simulink model "MotoTron_validation_IO_model_integration"  (R2018a)
settings: Solver=FixedStepDiscrete  StartTime=0.0  StopTime=10.0  RelTol=1e-3  EnableMultiTasking=on
undefined symbols (not defined in the file or in its folder): ECU565, motohawk_build_version, motohawk_trunc_name, motohawk_vardec_path
libraries: MotoHawk_lib x73, simulink x16, motohawk_examples_lib x1
(part 2 of 2)

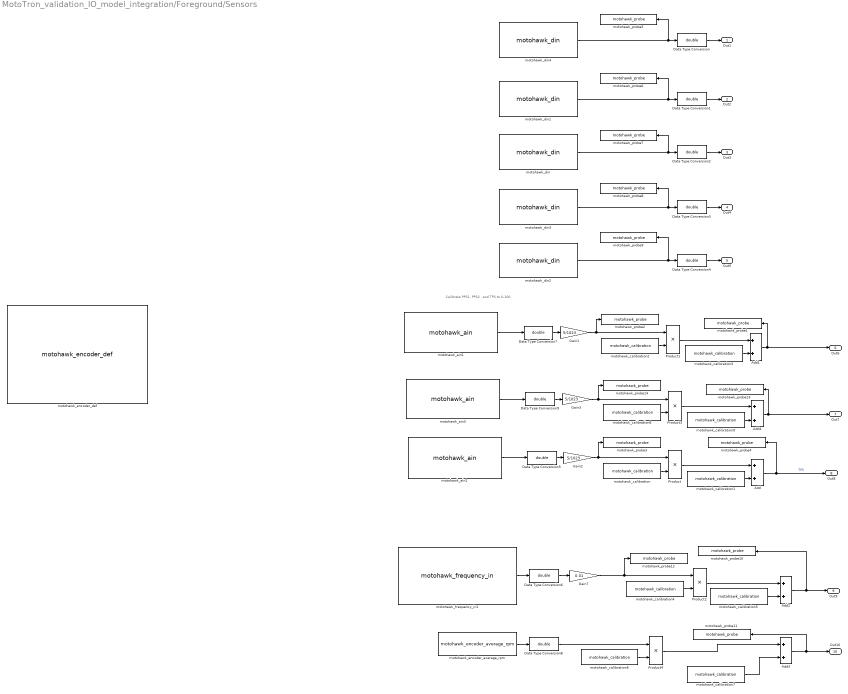
== system MotoTron_validation_IO_model_integration/Foreground/Sensors ==
  note: Calibrate PPS1, PPS2 , and TPS to 0-100
  Add{,1..4} (5 alike) : Sum
  Data Type Conversion{,1..9} (10 alike) : DataTypeConversion  OutDataTypeStr=double
  Gain1 : Gain  Gain=5/1023
  Gain2 : Gain  Gain=5/1023
  Gain3 : Gain  Gain=5/1023
  Gain7 : Gain  Gain=0.01
  Product{,1..4} (5 alike) : Product  RndMeth=Zero
  motohawk_ain1 : MotoHawk_lib/Analog I//O Blocks/motohawk_ain  res_name='PPS1'  text_resource=AN2M  code_resource=NONE  val_resource=-1  target=ECU565-128  resource_enum_str=(None)=-1,ECUP=53,DRVP=54,XDRP=55,AN1M=56,AN2M=57,AN3M=58,AN4M=59,AN5M=60,AN6M=61,AN7M=62,AN8M=63,AN9M=64,AN10M=65,AN11M=66,AN12M=67,AN13M=68,AN14M=69,AN15M=70,AN16M=71,AN17M=72,AN18M=73,AN19M=74,AN20M=75,AN21M=76,AN22M=77,AN23M=78,AN24M=79,AN25M=80,AN26M=81,AN27M=82,AN28M=83,AN29M=84,AN30M=85,AN31M=86,AN32M=87,AN33M=88,AN34M=89,O2A=90,O2B=91,XDRP_B=92,REF_14V=143  altref=5V Reference  typ=uint16  num_adc_bits=10  use_stat=off  use_vardec=off  nam='RTD1_MW'  read_level=1  write_level=1  group='System | I/O Pins | Inputs Config'
      settings: SourceProductName=MotoHawk
  motohawk_ain2 : MotoHawk_lib/Analog I//O Blocks/motohawk_ain  res_name='TPS'  text_resource=AN4M  code_resource=NONE  val_resource=-1  target=ECU565-128  resource_enum_str=(None)=-1,ECUP=53,DRVP=54,XDRP=55,AN1M=56,AN2M=57,AN3M=58,AN4M=59,AN5M=60,AN6M=61,AN7M=62,AN8M=63,AN9M=64,AN10M=65,AN11M=66,AN12M=67,AN13M=68,AN14M=69,AN15M=70,AN16M=71,AN17M=72,AN18M=73,AN19M=74,AN20M=75,AN21M=76,AN22M=77,AN23M=78,AN24M=79,AN25M=80,AN26M=81,AN27M=82,AN28M=83,AN29M=84,AN30M=85,AN31M=86,AN32M=87,AN33M=88,AN34M=89,O2A=90,O2B=91,XDRP_B=92,REF_14V=143  altref=5V Reference  typ=uint16  num_adc_bits=10  use_stat=off  use_vardec=off  nam='RTD1_MW'  read_level=1  write_level=1  group='System | I/O Pins | Inputs Config'
      settings: SourceProductName=MotoHawk
  motohawk_ain3 : MotoHawk_lib/Analog I//O Blocks/motohawk_ain  res_name='PPS2'  text_resource=AN3M  code_resource=NONE  val_resource=-1  target=ECU565-128  resource_enum_str=(None)=-1,ECUP=53,DRVP=54,XDRP=55,AN1M=56,AN2M=57,AN3M=58,AN4M=59,AN5M=60,AN6M=61,AN7M=62,AN8M=63,AN9M=64,AN10M=65,AN11M=66,AN12M=67,AN13M=68,AN14M=69,AN15M=70,AN16M=71,AN17M=72,AN18M=73,AN19M=74,AN20M=75,AN21M=76,AN22M=77,AN23M=78,AN24M=79,AN25M=80,AN26M=81,AN27M=82,AN28M=83,AN29M=84,AN30M=85,AN31M=86,AN32M=87,AN33M=88,AN34M=89,O2A=90,O2B=91,XDRP_B=92,REF_14V=143  altref=5V Reference  typ=uint16  num_adc_bits=10  use_stat=off  use_vardec=off  nam='RTD1_MW'  read_level=1  write_level=1  group='System | I/O Pins | Inputs Config'
      settings: SourceProductName=MotoHawk
  motohawk_calibration : MotoHawk_lib/Calibration & Probing Blocks/motohawk_calibration  nam='TPS_Gain'  val=1  storage=Calibration  show_more=on  name_source=Use Parameter  data_type=Inherit from 'Default Value'  read_level=1  write_level=1  ovr_cals=off  view_as=Number  enum_struct={'Disabled', 'Enabled'}  vector_style=Wide Row  use_help_units=off  help=''  units=''  use_header_enum=off  row_header_enum={}  col_header_enum={}  use_min_max=off  min_val=-inf  max_val=inf  use_precision=off  precision=''  gain=1  offset=0  exp=1  use_mototune_group=off  mototune_group=motohawk_vardec_path(gcb)  data_stores=motohawk_sfun_calibration_data_stores
      settings: SourceProductName=MotoHawk
  motohawk_calibration1 : MotoHawk_lib/Calibration & Probing Blocks/motohawk_calibration  nam='TPS_Offset'  val=0  storage=Calibration  show_more=on  name_source=Use Parameter  data_type=Inherit from 'Default Value'  read_level=1  write_level=1  ovr_cals=off  view_as=Number  enum_struct={'Disabled', 'Enabled'}  vector_style=Wide Row  use_help_units=off  help=''  units=''  use_header_enum=off  row_header_enum={}  col_header_enum={}  use_min_max=off  min_val=-inf  max_val=inf  use_precision=off  precision=''  gain=1  offset=0  exp=1  use_mototune_group=off  mototune_group=motohawk_vardec_path(gcb)  data_stores=motohawk_sfun_calibration_data_stores
      settings: SourceProductName=MotoHawk
  motohawk_calibration2 : MotoHawk_lib/Calibration & Probing Blocks/motohawk_calibration  nam='PPS1_Gain'  val=1  storage=Calibration  show_more=on  name_source=Use Parameter  data_type=Inherit from 'Default Value'  read_level=1  write_level=1  ovr_cals=off  view_as=Number  enum_struct={'Disabled', 'Enabled'}  vector_style=Wide Row  use_help_units=off  help=''  units=''  use_header_enum=off  row_header_enum={}  col_header_enum={}  use_min_max=off  min_val=-inf  max_val=inf  use_precision=off  precision=''  gain=1  offset=0  exp=1  use_mototune_group=off  mototune_group=motohawk_vardec_path(gcb)  data_stores=motohawk_sfun_calibration_data_stores
      settings: SourceProductName=MotoHawk
  motohawk_calibration3 : MotoHawk_lib/Calibration & Probing Blocks/motohawk_calibration  nam='PPS1_Offset'  val=0  storage=Calibration  show_more=on  name_source=Use Parameter  data_type=Inherit from 'Default Value'  read_level=1  write_level=1  ovr_cals=off  view_as=Number  enum_struct={'Disabled', 'Enabled'}  vector_style=Wide Row  use_help_units=off  help=''  units=''  use_header_enum=off  row_header_enum={}  col_header_enum={}  use_min_max=off  min_val=-inf  max_val=inf  use_precision=off  precision=''  gain=1  offset=0  exp=1  use_mototune_group=off  mototune_group=motohawk_vardec_path(gcb)  data_stores=motohawk_sfun_calibration_data_stores
      settings: SourceProductName=MotoHawk
  motohawk_calibration4 : MotoHawk_lib/Calibration & Probing Blocks/motohawk_calibration  nam='Vehicle_Speed_Gain'  val=1  storage=Calibration  show_more=on  name_source=Use Parameter  data_type=Inherit from 'Default Value'  read_level=1  write_level=1  ovr_cals=off  view_as=Number  enum_struct={'Disabled', 'Enabled'}  vector_style=Wide Row  use_help_units=off  help=''  units=''  use_header_enum=off  row_header_enum={}  col_header_enum={}  use_min_max=off  min_val=-inf  max_val=inf  use_precision=off  precision=''  gain=1  offset=0  exp=1  use_mototune_group=off  mototune_group=motohawk_vardec_path(gcb)  data_stores=motohawk_sfun_calibration_data_stores
      settings: SourceProductName=MotoHawk
  motohawk_calibration5 : MotoHawk_lib/Calibration & Probing Blocks/motohawk_calibration  nam='Vehicle_Speed_Offset'  val=0  storage=Calibration  show_more=on  name_source=Use Parameter  data_type=Inherit from 'Default Value'  read_level=1  write_level=1  ovr_cals=off  view_as=Number  enum_struct={'Disabled', 'Enabled'}  vector_style=Wide Row  use_help_units=off  help=''  units=''  use_header_enum=off  row_header_enum={}  col_header_enum={}  use_min_max=off  min_val=-inf  max_val=inf  use_precision=off  precision=''  gain=1  offset=0  exp=1  use_mototune_group=off  mototune_group=motohawk_vardec_path(gcb)  data_stores=motohawk_sfun_calibration_data_stores
      settings: SourceProductName=MotoHawk
  motohawk_calibration6 : MotoHawk_lib/Calibration & Probing Blocks/motohawk_calibration  nam='Engine_RPM_Gain'  val=1  storage=Calibration  show_more=on  name_source=Use Parameter  data_type=Inherit from 'Default Value'  read_level=1  write_level=1  ovr_cals=off  view_as=Number  enum_struct={'Disabled', 'Enabled'}  vector_style=Wide Row  use_help_units=off  help=''  units=''  use_header_enum=off  row_header_enum={}  col_header_enum={}  use_min_max=off  min_val=-inf  max_val=inf  use_precision=off  precision=''  gain=1  offset=0  exp=1  use_mototune_group=off  mototune_group=motohawk_vardec_path(gcb)  data_stores=motohawk_sfun_calibration_data_stores
      settings: SourceProductName=MotoHawk
  motohawk_calibration7 : MotoHawk_lib/Calibration & Probing Blocks/motohawk_calibration  nam='Engine_RPM_Offset'  val=0  storage=Calibration  show_more=on  name_source=Use Parameter  data_type=Inherit from 'Default Value'  read_level=1  write_level=1  ovr_cals=off  view_as=Number  enum_struct={'Disabled', 'Enabled'}  vector_style=Wide Row  use_help_units=off  help=''  units=''  use_header_enum=off  row_header_enum={}  col_header_enum={}  use_min_max=off  min_val=-inf  max_val=inf  use_precision=off  precision=''  gain=1  offset=0  exp=1  use_mototune_group=off  mototune_group=motohawk_vardec_path(gcb)  data_stores=motohawk_sfun_calibration_data_stores
      settings: SourceProductName=MotoHawk
  motohawk_calibration8 : MotoHawk_lib/Calibration & Probing Blocks/motohawk_calibration  nam='PPS2_Gain'  val=1  storage=Calibration  show_more=on  name_source=Use Parameter  data_type=Inherit from 'Default Value'  read_level=1  write_level=1  ovr_cals=off  view_as=Number  enum_struct={'Disabled', 'Enabled'}  vector_style=Wide Row  use_help_units=off  help=''  units=''  use_header_enum=off  row_header_enum={}  col_header_enum={}  use_min_max=off  min_val=-inf  max_val=inf  use_precision=off  precision=''  gain=1  offset=0  exp=1  use_mototune_group=off  mototune_group=motohawk_vardec_path(gcb)  data_stores=motohawk_sfun_calibration_data_stores
      settings: SourceProductName=MotoHawk
  motohawk_calibration9 : MotoHawk_lib/Calibration & Probing Blocks/motohawk_calibration  nam='PPS2_Offset'  val=0  storage=Calibration  show_more=on  name_source=Use Parameter  data_type=Inherit from 'Default Value'  read_level=1  write_level=1  ovr_cals=off  view_as=Number  enum_struct={'Disabled', 'Enabled'}  vector_style=Wide Row  use_help_units=off  help=''  units=''  use_header_enum=off  row_header_enum={}  col_header_enum={}  use_min_max=off  min_val=-inf  max_val=inf  use_precision=off  precision=''  gain=1  offset=0  exp=1  use_mototune_group=off  mototune_group=motohawk_vardec_path(gcb)  data_stores=motohawk_sfun_calibration_data_stores
      settings: SourceProductName=MotoHawk
  motohawk_din : MotoHawk_lib/Digital I//O Blocks/motohawk_din  resource_name='Motor_On_Switch'  text_resource=AN6M  code_resource=NONE  val_resource=-1  target=ECU565-128  resource_enum_str=(None)=-1,AN1M=56,AN2M=57,AN3M=58,AN4M=59,AN5M=60,AN6M=61,AN7M=62,AN8M=63,AN9M=64,AN10M=65,AN11M=66,AN12M=67,AN13M=68,AN14M=69,AN15M=70,AN16M=71,AN17M=72,AN18M=73,AN19M=74,AN20M=75,AN21M=76,AN22M=77,AN23M=78,AN24M=79,AN25M=80,AN26M=81,AN27M=82,AN28M=83,AN29M=84,AN30M=85,AN31M=86,AN32M=87,AN33M=88,AN34M=89,O2A=90,O2B=91,DG1M=93,DG2M=94,DG3M=95,DG4M=96,DG5M=102,DG6M=103,DG7M=104,SPD1=105,SPD2=106,DG8M=111  pullup=Strong  use_stat=off  use_vardec=off  nam='DIN'  read_level=1  write_level=1  group='System | I/O Pins | Inputs Config'
      settings: SourceProductName=MotoHawk
  motohawk_din1 : MotoHawk_lib/Digital I//O Blocks/motohawk_din  resource_name='Engine_On_Switch'  text_resource=AN5M  code_resource=NONE  val_resource=-1  target=ECU565-128  resource_enum_str=(None)=-1,AN1M=56,AN2M=57,AN3M=58,AN4M=59,AN5M=60,AN6M=61,AN7M=62,AN8M=63,AN9M=64,AN10M=65,AN11M=66,AN12M=67,AN13M=68,AN14M=69,AN15M=70,AN16M=71,AN17M=72,AN18M=73,AN19M=74,AN20M=75,AN21M=76,AN22M=77,AN23M=78,AN24M=79,AN25M=80,AN26M=81,AN27M=82,AN28M=83,AN29M=84,AN30M=85,AN31M=86,AN32M=87,AN33M=88,AN34M=89,O2A=90,O2B=91,DG1M=93,DG2M=94,DG3M=95,DG4M=96,DG5M=102,DG6M=103,DG7M=104,SPD1=105,SPD2=106,DG8M=111  pullup=Strong  use_stat=off  use_vardec=off  nam='DIN'  read_level=1  write_level=1  group='System | I/O Pins | Inputs Config'
      settings: SourceProductName=MotoHawk
  motohawk_din2 : MotoHawk_lib/Digital I//O Blocks/motohawk_din  resource_name='Reverse_Switch'  text_resource=AN8M  code_resource=NONE  val_resource=-1  target=ECU565-128  resource_enum_str=(None)=-1,AN1M=56,AN2M=57,AN3M=58,AN4M=59,AN5M=60,AN6M=61,AN7M=62,AN8M=63,AN9M=64,AN10M=65,AN11M=66,AN12M=67,AN13M=68,AN14M=69,AN15M=70,AN16M=71,AN17M=72,AN18M=73,AN19M=74,AN20M=75,AN21M=76,AN22M=77,AN23M=78,AN24M=79,AN25M=80,AN26M=81,AN27M=82,AN28M=83,AN29M=84,AN30M=85,AN31M=86,AN32M=87,AN33M=88,AN34M=89,O2A=90,O2B=91,DG1M=93,DG2M=94,DG3M=95,DG4M=96,DG5M=102,DG6M=103,DG7M=104,SPD1=105,SPD2=106,DG8M=111  pullup=Strong  use_stat=off  use_vardec=off  nam='DIN'  read_level=1  write_level=1  group='System | I/O Pins | Inputs Config'
      settings: SourceProductName=MotoHawk
  motohawk_din3 : MotoHawk_lib/Digital I//O Blocks/motohawk_din  resource_name='Forward_Switch'  text_resource=AN7M  code_resource=NONE  val_resource=-1  target=ECU565-128  resource_enum_str=(None)=-1,AN1M=56,AN2M=57,AN3M=58,AN4M=59,AN5M=60,AN6M=61,AN7M=62,AN8M=63,AN9M=64,AN10M=65,AN11M=66,AN12M=67,AN13M=68,AN14M=69,AN15M=70,AN16M=71,AN17M=72,AN18M=73,AN19M=74,AN20M=75,AN21M=76,AN22M=77,AN23M=78,AN24M=79,AN25M=80,AN26M=81,AN27M=82,AN28M=83,AN29M=84,AN30M=85,AN31M=86,AN32M=87,AN33M=88,AN34M=89,O2A=90,O2B=91,DG1M=93,DG2M=94,DG3M=95,DG4M=96,DG5M=102,DG6M=103,DG7M=104,SPD1=105,SPD2=106,DG8M=111  pullup=Strong  use_stat=off  use_vardec=off  nam='DIN'  read_level=1  write_level=1  group='System | I/O Pins | Inputs Config'
      settings: SourceProductName=MotoHawk
  motohawk_din4 : MotoHawk_lib/Digital I//O Blocks/motohawk_din  resource_name='Crank_Switch'  text_resource=AN9M  code_resource=NONE  val_resource=-1  target=ECU565-128  resource_enum_str=(None)=-1,AN1M=56,AN2M=57,AN3M=58,AN4M=59,AN5M=60,AN6M=61,AN7M=62,AN8M=63,AN9M=64,AN10M=65,AN11M=66,AN12M=67,AN13M=68,AN14M=69,AN15M=70,AN16M=71,AN17M=72,AN18M=73,AN19M=74,AN20M=75,AN21M=76,AN22M=77,AN23M=78,AN24M=79,AN25M=80,AN26M=81,AN27M=82,AN28M=83,AN29M=84,AN30M=85,AN31M=86,AN32M=87,AN33M=88,AN34M=89,O2A=90,O2B=91,DG1M=93,DG2M=94,DG3M=95,DG4M=96,DG5M=102,DG6M=103,DG7M=104,SPD1=105,SPD2=106,DG8M=111  pullup=Strong  use_stat=off  use_vardec=off  nam='DIN'  read_level=1  write_level=1  group='System | I/O Pins | Inputs Config'
      settings: SourceProductName=MotoHawk
  motohawk_encoder_average_rpm : MotoHawk_lib/Encoder Blocks/motohawk_encoder_average_rpm  resolution=1
      settings: SourceProductName=MotoHawk
  motohawk_encoder_def : MotoHawk_lib/Encoder Blocks/motohawk_encoder_def  encoder_type=36 Minus 1 - 4-Stroke - No CAM  interface=Digital Crank  sync=Falling Edge  crnkpullup=Weak Pullup  camsync=Rising Edge  campullup=Weak Pullup  angle_offset=0  sec_tdcoffset=0  cam_delay=0  teeth_after_cam=-1  ignore_teeth=0  ignore_delay=0  angles=[0 360 180 540]  cnk_align_with_cam=off  adaptive_vr_cnk=off  adaptive_vr_cam=on  cal_cylinders=on  max_cylinders=8  num_cylinders=1  read_level=1  write_level=1  ovr_cals=on  group='System | Encoder'
      settings: SourceProductName=MotoHawk
  motohawk_frequency_in1 : MotoHawk_lib/Advanced Digital I//O/motohawk_frequency_in  res_name='Vehicle_Speed'  text_resource=SPD1  code_resource=NONE  val_resource=-1  target=ECU565-128  resource_enum_str=(None)=-1,DG1M=93,DG2M=94,DG3M=95,DG4M=96,DG5M=102,DG6M=103,DG7M=104,SPD1=105,SPD2=106,DG8M=111  edge=Rising Edge  alias=Enabled  min_freq=0  sig=Digital Input  ipwm=No Duty Cycle Measurement  show_newness_status=off  itrig=off  Nmax=10  use_avg=off  avg_mode=Fixed Interval  fixed_avg_pulses=2  use_vardec=off  use_cal=off  nam='FreqInPin'  read_level=1  write_level=1  group='System | I/O Pins | Inputs Config'  cal_group='System | I/O Pins | Frequency In Config'
      settings: SourceProductName=MotoHawk
  motohawk_probe1 : MotoHawk_lib/Calibration & Probing Blocks/motohawk_probe  nam='PPS1'  show_more=off  name_source=Use Parameter  read_level=1  view_as=Number  enum_struct={'Disabled', 'Enabled'}  vector_style=Wide Row  use_help_units=off  help=''  units=''  use_header_enum=off  row_header_enum={}  col_header_enum={}  use_min_max=off  min_val=-inf  max_val=inf  use_precision=off  precision=''  gain=1  offset=0  exp=1  use_mototune_group=off  mototune_group=motohawk_vardec_path(gcb)
      settings: SourceProductName=MotoHawk
  motohawk_probe10 : MotoHawk_lib/Calibration & Probing Blocks/motohawk_probe  nam='Vehicle_Speed'  show_more=off  name_source=Use Parameter  read_level=1  view_as=Number  enum_struct={'Disabled', 'Enabled'}  vector_style=Wide Row  use_help_units=off  help=''  units=''  use_header_enum=off  row_header_enum={}  col_header_enum={}  use_min_max=off  min_val=-inf  max_val=inf  use_precision=off  precision=''  gain=1  offset=0  exp=1  use_mototune_group=off  mototune_group=motohawk_vardec_path(gcb)
      settings: SourceProductName=MotoHawk
  motohawk_probe11 : MotoHawk_lib/Calibration & Probing Blocks/motohawk_probe  nam='Engine_RPM'  show_more=off  name_source=Use Parameter  read_level=1  view_as=Number  enum_struct={'Disabled', 'Enabled'}  vector_style=Wide Row  use_help_units=off  help=''  units=''  use_header_enum=off  row_header_enum={}  col_header_enum={}  use_min_max=off  min_val=-inf  max_val=inf  use_precision=off  precision=''  gain=1  offset=0  exp=1  use_mototune_group=off  mototune_group=motohawk_vardec_path(gcb)
      settings: SourceProductName=MotoHawk
  motohawk_probe12 : MotoHawk_lib/Calibration & Probing Blocks/motohawk_probe  nam='Vehicle_Speed_beforeCalibration'  show_more=off  name_source=Use Parameter  read_level=1  view_as=Number  enum_struct={'Disabled', 'Enabled'}  vector_style=Wide Row  use_help_units=off  help=''  units=''  use_header_enum=off  row_header_enum={}  col_header_enum={}  use_min_max=off  min_val=-inf  max_val=inf  use_precision=off  precision=''  gain=1  offset=0  exp=1  use_mototune_group=off  mototune_group=motohawk_vardec_path(gcb)
      settings: SourceProductName=MotoHawk
  motohawk_probe13 : MotoHawk_lib/Calibration & Probing Blocks/motohawk_probe  nam='PPS2'  show_more=off  name_source=Use Parameter  read_level=1  view_as=Number  enum_struct={'Disabled', 'Enabled'}  vector_style=Wide Row  use_help_units=off  help=''  units=''  use_header_enum=off  row_header_enum={}  col_header_enum={}  use_min_max=off  min_val=-inf  max_val=inf  use_precision=off  precision=''  gain=1  offset=0  exp=1  use_mototune_group=off  mototune_group=motohawk_vardec_path(gcb)
      settings: SourceProductName=MotoHawk
  motohawk_probe14 : MotoHawk_lib/Calibration & Probing Blocks/motohawk_probe  nam='PPS2_beforeCalibration'  show_more=off  name_source=Use Parameter  read_level=1  view_as=Number  enum_struct={'Disabled', 'Enabled'}  vector_style=Wide Row  use_help_units=off  help=''  units=''  use_header_enum=off  row_header_enum={}  col_header_enum={}  use_min_max=off  min_val=-inf  max_val=inf  use_precision=off  precision=''  gain=1  offset=0  exp=1  use_mototune_group=off  mototune_group=motohawk_vardec_path(gcb)
      settings: SourceProductName=MotoHawk
  motohawk_probe2 : MotoHawk_lib/Calibration & Probing Blocks/motohawk_probe  nam='PPS1_beforeCalibration'  show_more=off  name_source=Use Parameter  read_level=1  view_as=Number  enum_struct={'Disabled', 'Enabled'}  vector_style=Wide Row  use_help_units=off  help=''  units=''  use_header_enum=off  row_header_enum={}  col_header_enum={}  use_min_max=off  min_val=-inf  max_val=inf  use_precision=off  precision=''  gain=1  offset=0  exp=1  use_mototune_group=off  mototune_group=motohawk_vardec_path(gcb)
      settings: SourceProductName=MotoHawk
  motohawk_probe3 : MotoHawk_lib/Calibration & Probing Blocks/motohawk_probe  nam='TPS_beforeCalibration'  show_more=on  name_source=Use Parameter  read_level=1  view_as=Number  enum_struct={'Disabled', 'Enabled'}  vector_style=Wide Row  use_help_units=off  help=''  units=''  use_header_enum=off  row_header_enum={}  col_header_enum={}  use_min_max=off  min_val=-inf  max_val=inf  use_precision=off  precision=''  gain=1  offset=0  exp=1  use_mototune_group=off  mototune_group=motohawk_vardec_path(gcb)
      settings: SourceProductName=MotoHawk
  motohawk_probe4 : MotoHawk_lib/Calibration & Probing Blocks/motohawk_probe  nam='TPS'  show_more=off  name_source=Use Parameter  read_level=1  view_as=Number  enum_struct={'Disabled', 'Enabled'}  vector_style=Wide Row  use_help_units=off  help=''  units=''  use_header_enum=off  row_header_enum={}  col_header_enum={}  use_min_max=off  min_val=-inf  max_val=inf  use_precision=off  precision=''  gain=1  offset=0  exp=1  use_mototune_group=off  mototune_group=motohawk_vardec_path(gcb)
      settings: SourceProductName=MotoHawk
  motohawk_probe5 : MotoHawk_lib/Calibration & Probing Blocks/motohawk_probe  nam='Crank_Switch'  show_more=off  name_source=Use Parameter  read_level=1  view_as=Number  enum_struct={'Disabled', 'Enabled'}  vector_style=Wide Row  use_help_units=off  help=''  units=''  use_header_enum=off  row_header_enum={}  col_header_enum={}  use_min_max=off  min_val=-inf  max_val=inf  use_precision=off  precision=''  gain=1  offset=0  exp=1  use_mototune_group=off  mototune_group=motohawk_vardec_path(gcb)
      settings: SourceProductName=MotoHawk
  motohawk_probe6 : MotoHawk_lib/Calibration & Probing Blocks/motohawk_probe  nam='Engine_On_Switch'  show_more=off  name_source=Use Parameter  read_level=1  view_as=Number  enum_struct={'Disabled', 'Enabled'}  vector_style=Wide Row  use_help_units=off  help=''  units=''  use_header_enum=off  row_header_enum={}  col_header_enum={}  use_min_max=off  min_val=-inf  max_val=inf  use_precision=off  precision=''  gain=1  offset=0  exp=1  use_mototune_group=off  mototune_group=motohawk_vardec_path(gcb)
      settings: SourceProductName=MotoHawk
  motohawk_probe7 : MotoHawk_lib/Calibration & Probing Blocks/motohawk_probe  nam='Motor_On_Switch'  show_more=off  name_source=Use Parameter  read_level=1  view_as=Number  enum_struct={'Disabled', 'Enabled'}  vector_style=Wide Row  use_help_units=off  help=''  units=''  use_header_enum=off  row_header_enum={}  col_header_enum={}  use_min_max=off  min_val=-inf  max_val=inf  use_precision=off  precision=''  gain=1  offset=0  exp=1  use_mototune_group=off  mototune_group=motohawk_vardec_path(gcb)
      settings: SourceProductName=MotoHawk
  motohawk_probe8 : MotoHawk_lib/Calibration & Probing Blocks/motohawk_probe  nam='Foward_Switch'  show_more=off  name_source=Use Parameter  read_level=1  view_as=Number  enum_struct={'Disabled', 'Enabled'}  vector_style=Wide Row  use_help_units=off  help=''  units=''  use_header_enum=off  row_header_enum={}  col_header_enum={}  use_min_max=off  min_val=-inf  max_val=inf  use_precision=off  precision=''  gain=1  offset=0  exp=1  use_mototune_group=off  mototune_group=motohawk_vardec_path(gcb)
      settings: SourceProductName=MotoHawk
  motohawk_probe9 : MotoHawk_lib/Calibration & Probing Blocks/motohawk_probe  nam='Reverse_Switch'  show_more=off  name_source=Use Parameter  read_level=1  view_as=Number  enum_struct={'Disabled', 'Enabled'}  vector_style=Wide Row  use_help_units=off  help=''  units=''  use_header_enum=off  row_header_enum={}  col_header_enum={}  use_min_max=off  min_val=-inf  max_val=inf  use_precision=off  precision=''  gain=1  offset=0  exp=1  use_mototune_group=off  mototune_group=motohawk_vardec_path(gcb)
      settings: SourceProductName=MotoHawk
  Out1 : Outport
  Out2 : Outport  Port=2
  Out3 : Outport  Port=3
  Out4 : Outport  Port=4
  Out5 : Outport  Port=5
  Out6 : Outport  Port=6
  Out7 : Outport  Port=7
  Out8 : Outport  Port=8
  Out9 : Outport  Port=9
  Out10 : Outport  Port=10
  wires:
  Add4/1 -> Out7/1, motohawk_probe13/1
  Product3/1 -> Add4/1
  Gain3/1 -> Product3/1, motohawk_probe14/1
  motohawk_ain3/1 -> Data Type Conversion9/1
  motohawk_calibration9/1 -> Add4/2
  motohawk_calibration8/1 -> Product3/2
  motohawk_din1/1 -> motohawk_probe6/1, Data Type Conversion1/1
  motohawk_calibration7/1 -> Add3/2
  Data Type Conversion6/1 -> Gain7/1
  Gain1/1 -> Product1/1, motohawk_probe2/1
  Gain2/1 -> motohawk_probe3/1, Product/1
  Add3/1 -> motohawk_probe11/1, Out10/1
  motohawk_frequency_in1/1 -> Data Type Conversion6/1
  Data Type Conversion4/1 -> Out5/1
  motohawk_din4/1 -> motohawk_probe5/1, Data Type Conversion/1
  Data Type Conversion1/1 -> Out2/1
  Data Type Conversion/1 -> Out1/1
  Data Type Conversion3/1 -> Out4/1
  Data Type Conversion7/1 -> Gain1/1
  Add1/1 -> Out6/1, motohawk_probe1/1
  Data Type Conversion2/1 -> Out3/1
  motohawk_calibration4/1 -> Product2/2
  motohawk_calibration/1 -> Product/2
  motohawk_calibration5/1 -> Add2/2
  Product1/1 -> Add1/1
  Product2/1 -> Add2/1
  motohawk_din3/1 -> motohawk_probe8/1, Data Type Conversion3/1
  motohawk_ain2/1 -> Data Type Conversion5/1
  motohawk_ain1/1 -> Data Type Conversion7/1
  motohawk_calibration6/1 -> Product4/2
  motohawk_encoder_average_rpm/1 -> Data Type Conversion8/1
  motohawk_din/1 -> motohawk_probe7/1, Data Type Conversion2/1
  motohawk_calibration1/1 -> Add/2
  Data Type Conversion8/1 -> Product4/1
  Gain7/1 -> Product2/1, motohawk_probe12/1
  Add/1 -> motohawk_probe4/1, Out8/1  "TPS"
  Product4/1 -> Add3/1
  motohawk_calibration2/1 -> Product1/2
  motohawk_din2/1 -> motohawk_probe9/1, Data Type Conversion4/1
  Data Type Conversion5/1 -> Gain2/1
  Data Type Conversion9/1 -> Gain3/1
  Add2/1 -> Out9/1, motohawk_probe10/1
  Product/1 -> Add/1
  motohawk_calibration3/1 -> Add1/2

== stateflow chart MotoTron_validation_IO_model_integration/Foreground/Engine State  ==
  state Engine_State_Logic
    state Engineoffstate
      entry:
      engine_state=1;
    state EngineCrankState
      during:
      engine_state=2;
    state EngineWarmUp
      during:
      engine_state=3;
    state EngineOn
      during:
      engine_state=4;
    state EngineStartFail
      during:
      engine_state=5;
    (default) -> Engineoffstate
    EngineStartFail -> Engineoffstate
    Engineoffstate -> EngineCrankState : [crank ==1 && kill==0]
    EngineOn -> Engineoffstate : [RPM<50 || kill==1]
    EngineCrankState -> EngineWarmUp [order 1] : [RPM>800 && after(0.6,sec)]
    EngineCrankState -> EngineStartFail [order 2] : [RPM<=800 && after(1,sec)]
    EngineWarmUp -> EngineOn [order 1] : [RPM>=500 && after(1,sec)]
    EngineWarmUp -> EngineStartFail [order 2] : [RPM<500 && after(1,sec)]
  (default) -> Engine_State_Logic
  data: RPM input; kill input; crank input; engine_state output

== stateflow chart MotoTron_validation_IO_model_integration/Foreground/Chart1 ==
  state ThrottleRequest
    state intermediate
      during:
      enginetorquerequest=7.5;
    state Engine_Solo
      during:
      enginetorquerequest=APP;
    state Blending
      during:
      enginetorquerequest=APP*EngineBlendFactor;
      motortorquerequest=APP*MotorBlendFactor;
    state Electric_Solo
      during:
      motortorquerequest=APP;
    intermediate -> Blending [order 1] : [EngineState==4 && DrivingMode==2]
    Engine_Solo -> intermediate [order 1] : [EngineState==2 || EngineState==3 && DrivingMode==2 ]
    intermediate -> Engine_Solo [order 2] : [DrivingMode==3]
    Blending -> intermediate [order 1] : [EngineState==2 || EngineState==3 && DrivingMode==2]
    Engine_Solo -> Blending [order 2] : [EngineState==4 && DrivingMode==2]
    Engine_Solo -> Electric_Solo [order 3] : [DrivingMode==1]
    Electric_Solo -> Engine_Solo [order 1] : [DrivingMode==3]
    Blending -> Electric_Solo [order 2] : [DrivingMode==1]
    Electric_Solo -> Blending [order 2] : [DrivingMode==2]
    (default) -> Electric_Solo
  (default) -> ThrottleRequest
  data: EngineBlendFactor input; MotorBlendFactor input; DrivingMode input; EngineState input; APP input; enginetorquerequest output; motortorquerequest output

== stateflow chart MotoTron_validation_IO_model_integration/Foreground/Chart ==
  state Driving_Mode_Model
    state Electric_Solo
      entry:
      drive_mode=1;
    state Engine_Solo
      entry:
      drive_mode=3;
    state Blending_Mode
      entry:
      drive_mode=2;
    Electric_Solo -> Engine_Solo [order 2] : [velocity<1 && Eon==1 && mon==0 && SOC < 0.3]
    Engine_Solo -> Electric_Solo [order 1] : [velocity<1 && Eon==0 && mon==1 && SOC>=0.3]
    Electric_Solo -> Blending_Mode [order 1] : [velocity<1 && Eon==1 && mon==1 && SOC>=0.3]
    Blending_Mode -> Electric_Solo [order 1] : [velocity<1 && Eon==0 && mon==1 && SOC>=0.3]
    Blending_Mode -> Engine_Solo [order 2] : [velocity<1 && Eon==1 && mon==0 && SOC<0.3]
    Engine_Solo -> Blending_Mode [order 2] : [velocity<1 && Eon==1 && mon==1 && SOC>=0.3]
  (default) -> Electric_Solo
  data: Eon input; mon input; velocity input; drive_mode output; SOC input

== matlab function MotoTron_validation_IO_model_integration/Foreground/MATLAB Function ==
  data: engineblendfactor input; enginekill output; drivingmode input; Engine_State input; crankswitch input; enginecrank output
function [enginekill, enginecrank] = fcn(engineblendfactor, drivingmode, Engine_State, crankswitch)
if drivingmode==1
    enginekill=1;
elseif drivingmode==2
    if engineblendfactor>0.01
        enginekill=0;
    else
        enginekill=1;
    end
else
    enginekill=0;
end

if drivingmode==1
    manualcrank=0;
    enginecrank=manualcrank;
elseif drivingmode==2
    if engineblendfactor>0.01 && Engine_State==1
        autocrank=1;
        enginecrank=autocrank;
    else
        enginecrank=0;
    end
elseif drivingmode==3 && crankswitch==1
    manualcrank=1;
    enginecrank=manualcrank;
else
    enginecrank=0;
end
end

== matlab function MotoTron_validation_IO_model_integration/Foreground/MATLAB Function1 ==
  data: motorblendfactor input; emotoron output; drivingmode input; forwardswitch input; reverseswitch input; forward output; reverse output; autocrank output; motorkill output
function [emotoron, forward, reverse, autocrank,motorkill] = fcn(motorblendfactor, drivingmode, forwardswitch, reverseswitch)
if drivingmode==1
    emotoron=1;
elseif drivingmode==2
    if motorblendfactor>0.01
        emotoron=1;
    else
        emotoron=0;
    end
else
    emotoron=0;
end

if drivingmode==1
    if forwardswitch==1 && reverseswitch==0
        forward=1;
    else
        forward=0;
    end    
    if reverseswitch==1 && forwardswitch==0
        reverse=1;
    else
        reverse=0;
    end
    if reverseswitch==1 && forwardswitch==1
        motorkill=1;
        autocrank=motorkill;
    else
        motorkill=0;
        autocrank=0;
    end     
else
    forward=0;
    reverse=0;
    motorkill=0;
    autocrank=0;
end
end

== stateflow chart MotoTron_validation_IO_model_integration/Foreground/Chart2 ==
  state Driving_Mode_Model
    state Electric_Solo
      entry:
      drive_mode=1;
    state Engine_Solo
      during:
      drive_mode=3;
    state Blending_Mode
      during:
      drive_mode=2;
    Electric_Solo -> Engine_Solo [order 2] : [velocity<1 && Eon==1 && mon==0 || SOC<0.3 || autocrank==1]
    Engine_Solo -> Electric_Solo [order 1] : [velocity<1 && Eon==0 && mon==1 && SOC>=0.3]
    Blending_Mode -> Electric_Solo [order 1] : [velocity<1 && Eon==0 && mon==1 && SOC>=0.3]
    Electric_Solo -> Blending_Mode [order 1] : [velocity<1 && Eon==0 && mon==0 && SOC>=0.3]
    Blending_Mode -> Engine_Solo [order 2] : [velocity<1 && Eon==1 && mon==0 || SOC<0.3 || autocrank==1]
    Engine_Solo -> Blending_Mode [order 2] : [velocity<1 && Eon==0 && mon==0 && SOC>=0.3]
  (default) -> Electric_Solo
  data: Eon input; mon input; velocity input; drive_mode output; SOC input; autocrank input

== stateflow chart MotoTron_validation_IO_model_integration/Foreground/Chart3 ==
  state ThrottleRequest
    state intermediate
      during:
      enginetorquerequest=7.5;
      motortorquerequest = APP*MotorBlendFactor
    state Engine_Solo
      during:
      enginetorquerequest=APP;
      motortorquerequest=0;
    state Blending
      during:
      enginetorquerequest=APP*EngineBlendFactor;
      motortorquerequest=APP*MotorBlendFactor;
    state Electric_Solo
      during:
      motortorquerequest=APP;
      enginetorquerequest=0;
    Engine_Solo -> intermediate [order 1] : [EngineState==2 || EngineState==3 && DrivingMode==2 ]
    intermediate -> Blending [order 1] : [EngineState==4 && DrivingMode==2]
    intermediate -> Engine_Solo [order 2] : [DrivingMode==3]
    Blending -> intermediate [order 1] : [EngineState==2 || EngineState==3 && DrivingMode==2]
    Engine_Solo -> Blending [order 2] : [EngineState==4 && DrivingMode==2]
    Engine_Solo -> Electric_Solo [order 3] : [DrivingMode==1]
    Electric_Solo -> Engine_Solo [order 1] : [DrivingMode==3]
    Blending -> Engine_Solo [order 3] : [DrivingMode==3]
    Blending -> Electric_Solo [order 2] : [DrivingMode==1]
    Electric_Solo -> Blending [order 2] : [DrivingMode==2]
    (default) -> Electric_Solo
  (default) -> ThrottleRequest
  data: EngineBlendFactor input; MotorBlendFactor input; DrivingMode input; EngineState input; APP input; enginetorquerequest output; motortorquerequest output

== stateflow chart MotoTron_validation_IO_model_integration/Foreground/Engine State 1 ==
  state Engine_State_Logic
    state Engineoffstate
      during:
      engine_state=1;
    state EngineCrankState
      during:
      engine_state=2;
    state EngineWarmUp
      during:
      engine_state=3;
    state EngineOn
      during:
      engine_state=4;
    state EngineStartFail
      entry:
      engine_state=5;
    (default) -> Engineoffstate
    Engineoffstate -> EngineCrankState : [crank ==1 && kill==0]
    EngineStartFail -> Engineoffstate
    EngineOn -> Engineoffstate : [RPM<50 || kill==1]
    EngineCrankState -> EngineWarmUp [order 1] : [RPM>800 && after(0.6,sec)]
    EngineCrankState -> EngineStartFail [order 2] : [RPM<=800 && after(1,sec)]
    EngineWarmUp -> EngineOn [order 1] : [RPM>=500 && after(1,sec)]
    EngineWarmUp -> EngineStartFail [order 2] : [RPM<500 && after(1,sec)]
  (default) -> Engine_State_Logic
  data: RPM input; kill input; crank input; engine_state output

== matlab function MotoTron_validation_IO_model_integration/Foreground/MATLAB Function2 ==
  data: engineblendfactor input; enginekill output; drivingmode input; Engine_State input; crankswitch input; enginecrank output; auto_crank output
function [enginekill, enginecrank,auto_crank] = fcn(engineblendfactor, drivingmode, Engine_State, crankswitch)
if drivingmode==1
    enginekill=1;
elseif drivingmode==2
    if engineblendfactor>0.01
        enginekill=0;
    else
        enginekill=1;
    end
else
    enginekill=0;
end

if drivingmode==1
    manualcrank=0;
    enginecrank=manualcrank;
    auto_crank=0;
elseif drivingmode==2
    if engineblendfactor>0.01 && Engine_State==1
        auto_crank=1;
        enginecrank=auto_crank;
    else
        enginecrank=0;
        auto_crank=0;
    end
elseif drivingmode==3 && crankswitch==1
    manualcrank=1;
    enginecrank=manualcrank;
    auto_crank = 0;
else
    enginecrank=0;
    auto_crank=0;
end
end

== matlab function MotoTron_validation_IO_model_integration/Foreground/MATLAB Function3 ==
  data: motorblendfactor input; emotoron output; drivingmode input; forwardswitch input; reverseswitch input; forward output; reverse output; autocrank output; motorkill output
function [emotoron, forward, reverse, autocrank,motorkill] = fcn(motorblendfactor, drivingmode, forwardswitch, reverseswitch)
if drivingmode==1
    emotoron=1;
elseif drivingmode==2
    if motorblendfactor>0.01
        emotoron=1;
    else
        emotoron=0;
    end
else
    emotoron=0;
end

if drivingmode==1
    if forwardswitch==1 && reverseswitch==0
        forward=1;
        reverse=0;
    elseif forwardswitch==0 && reverseswitch==1
        forward=0;
        reverse=1;
    else
        forward=0;
        reverse=0;
    end    
elseif drivingmode==2
        forward=1;
        reverse=0;
else
    forward=0;
    reverse=0;
end    
if reverseswitch==1 && forwardswitch==1
        motorkill=1;
        autocrank=motorkill;
else
        motorkill=0;
        autocrank=0;
end
end
